simulink model "con_retraso"  (R2018a)
settings: Solver=VariableStepAuto  StartTime=0.0  StopTime=10.0  RelTol=1e-3
settings Model: Creator=root  LastModifiedBy=root
settings DebuggingCC: LibraryContextMissingDiagnostic=warning
settings SFSimCC: SimUseLocalCustomCode=on
settings RTWCC: RTWUseLocalCustomCode=on

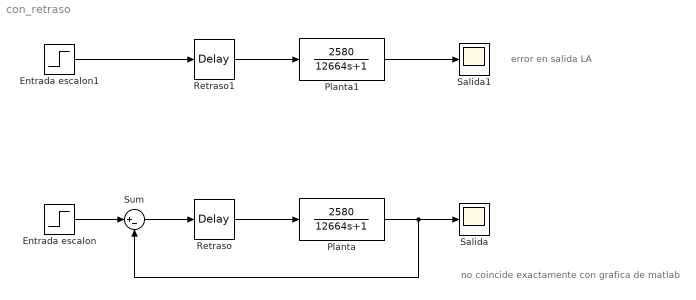
== system con_retraso ==
  note: no coincide exactamente con grafica de matlab
  note: error en salida LA
  Entrada escalon : Step  Time=0  SampleTime=0
  Entrada escalon1 : Step  Time=0  SampleTime=0
  Planta : TransferFcn  Numerator=[2580]  Denominator=[12664 1]
  Planta1 : TransferFcn  Numerator=[2580]  Denominator=[12664 1]
  Retraso : TransportDelay  DelayTime=2.1
  Retraso1 : TransportDelay  DelayTime=2.1
  Salida : Scope
  Salida1 : Scope
  Sum : Sum  Inputs=|+-
  wires:
  Entrada escalon/1 -> Sum/1
  Planta/1 -> Sum/2, Salida/1
  Sum/1 -> Retraso/1
  Retraso/1 -> Planta/1
  Retraso1/1 -> Planta1/1
  Planta1/1 -> Salida1/1
  Entrada escalon1/1 -> Retraso1/1
